simulink model "k1visproto"  (Simulink 8.2)
settings: Solver=ode45  StartTime=0.0  StopTime=10.0  RelTol=1e-3
libraries: cdsFiltCtrl x82, cdsFilt x45, cdsMuxMatrix x18, cdsEpicsOut x7, cdsEpicsBinIn x2, cdsAdcx0 x1, cdsAdcx1 x1, dac x1, simulink x1, cdsParameters x1
(part 14 of 14)

== system k1visproto/PROTO/TM/SERVOF ==
  L_IN : Inport
  P_IN : Inport  Port=2
  Y_IN : Inport  Port=3
  Ground1 : Ground
  Ground5 : Ground
  Ground6 : Ground
  L : cdsFiltCtrl/IIR FM with control  Tag=cdsFiltCtrl  Description=|
      | cdsFiltCntrl is the standard IIR filter module (exactly the same as cdsFilt) but with added control data output 'Ctrl'. Filter module digital signal output appears on the first output, which is called 'Val'. 'Ctrl' output has a bit pattern encoding the state of filter's on/off switches (FM1 through FM10). The bit values are:
      |                                                                                                                                                                                                                                                                                                                                       
      | module 	hex	dec                                                                                                                                                                                                                                                                                                                       
      | -----------------------                                                                                                                                                                                                                                                                                                               
      | FM1	0x20                    32                                                                                                                                                                                                                                                                                                        
      | FM2	0x80                     128                                                                                                                                                                                                                                                                                                      
      | FM3	0x200                   512                                                                                                                                                                                                                                                                                                       
      | FM4	0x800                   2048                                                                                                                                                                                                                                                                                                      
      | FM5	0x2000                 8192                                                                                                                                                                                                                                                                                                       
      | FM6	0x8000                 32768                                                                                                                                                                                                                                                                                                      
      | FM7	0x20000                131072                                                                                                                                                                                                                                                                                                     
      | FM8	0x80000                 524288                                                                                                                                                                                                                                                                                                    
      | FM9	0x200000               2097152                                                                                                                                                                                                                                                                                                    
      | FM10	0x800000               8388608                                                                                                                                                                                                                                                                                                   
      |                                                                                                                                                                                                                                                                                                                                       
      | This bit data can be used to drive some other switches or it can be output using a binary I/O module.
      settings: AttributesFormatString=%<Tag>
  P : cdsFiltCtrl/IIR FM with control  Tag=cdsFiltCtrl  Description=|
      | cdsFiltCntrl is the standard IIR filter module (exactly the same as cdsFilt) but with added control data output 'Ctrl'. Filter module digital signal output appears on the first output, which is called 'Val'. 'Ctrl' output has a bit pattern encoding the state of filter's on/off switches (FM1 through FM10). The bit values are:
      |                                                                                                                                                                                                                                                                                                                                       
      | module 	hex	dec                                                                                                                                                                                                                                                                                                                       
      | -----------------------                                                                                                                                                                                                                                                                                                               
      | FM1	0x20                    32                                                                                                                                                                                                                                                                                                        
      | FM2	0x80                     128                                                                                                                                                                                                                                                                                                      
      | FM3	0x200                   512                                                                                                                                                                                                                                                                                                       
      | FM4	0x800                   2048                                                                                                                                                                                                                                                                                                      
      | FM5	0x2000                 8192                                                                                                                                                                                                                                                                                                       
      | FM6	0x8000                 32768                                                                                                                                                                                                                                                                                                      
      | FM7	0x20000                131072                                                                                                                                                                                                                                                                                                     
      | FM8	0x80000                 524288                                                                                                                                                                                                                                                                                                    
      | FM9	0x200000               2097152                                                                                                                                                                                                                                                                                                    
      | FM10	0x800000               8388608                                                                                                                                                                                                                                                                                                   
      |                                                                                                                                                                                                                                                                                                                                       
      | This bit data can be used to drive some other switches or it can be output using a binary I/O module.
      settings: AttributesFormatString=%<Tag>
  Terminator1 : Terminator
  Terminator5 : Terminator
  Terminator6 : Terminator
  Y : cdsFiltCtrl/IIR FM with control  Tag=cdsFiltCtrl  Description=|
      | cdsFiltCntrl is the standard IIR filter module (exactly the same as cdsFilt) but with added control data output 'Ctrl'. Filter module digital signal output appears on the first output, which is called 'Val'. 'Ctrl' output has a bit pattern encoding the state of filter's on/off switches (FM1 through FM10). The bit values are:
      |                                                                                                                                                                                                                                                                                                                                       
      | module 	hex	dec                                                                                                                                                                                                                                                                                                                       
      | -----------------------                                                                                                                                                                                                                                                                                                               
      | FM1	0x20                    32                                                                                                                                                                                                                                                                                                        
      | FM2	0x80                     128                                                                                                                                                                                                                                                                                                      
      | FM3	0x200                   512                                                                                                                                                                                                                                                                                                       
      | FM4	0x800                   2048                                                                                                                                                                                                                                                                                                      
      | FM5	0x2000                 8192                                                                                                                                                                                                                                                                                                       
      | FM6	0x8000                 32768                                                                                                                                                                                                                                                                                                      
      | FM7	0x20000                131072                                                                                                                                                                                                                                                                                                     
      | FM8	0x80000                 524288                                                                                                                                                                                                                                                                                                    
      | FM9	0x200000               2097152                                                                                                                                                                                                                                                                                                    
      | FM10	0x800000               8388608                                                                                                                                                                                                                                                                                                   
      |                                                                                                                                                                                                                                                                                                                                       
      | This bit data can be used to drive some other switches or it can be output using a binary I/O module.
      settings: AttributesFormatString=%<Tag>
  L_Out : Outport
  P_Out : Outport  Port=2
  Y_Out : Outport  Port=3
  wires:
  Y/1 -> Y_Out/1
  P/1 -> P_Out/1
  Y_IN/1 -> Y/1
  Ground6/1 -> Y/2
  Y/2 -> Terminator6/1
  P_IN/1 -> P/1
  Ground5/1 -> P/2
  P/2 -> Terminator5/1
  L/1 -> L_Out/1
  L_IN/1 -> L/1
  Ground1/1 -> L/2
  L/2 -> Terminator1/1

== system k1visproto/PROTO/TM/TEST ==
  Ground1 : Ground
  Ground5 : Ground
  Ground6 : Ground
  L : cdsFilt/Subsystem  Tag=cdsFilt  Description=|
      | Purpose:                                                                                                                                                                                                                                  
      | Standard CDS IIR filter module.                                                                                                                                                                                                           
      |                                                                                                                                                                                                                                           
      | Operation:                                                                                                                                                                                                                                
      | Consists of 10 second order section IIR filters, plus a ramped gain stage. In FE code, also provides pre-defined test points and excitation channel inputs. The filter coefficients are defined in the LIGO system using the 'foton' tool.
      |                                                                                                                                                                                                                                           
      | Usage:                                                                                                                                                                                                                                    
      | Name the part with the desired filter module name.
      settings: AttributesFormatString=%<Tag>
  P : cdsFilt/Subsystem  Tag=cdsFilt  Description=|
      | Purpose:                                                                                                                                                                                                                                  
      | Standard CDS IIR filter module.                                                                                                                                                                                                           
      |                                                                                                                                                                                                                                           
      | Operation:                                                                                                                                                                                                                                
      | Consists of 10 second order section IIR filters, plus a ramped gain stage. In FE code, also provides pre-defined test points and excitation channel inputs. The filter coefficients are defined in the LIGO system using the 'foton' tool.
      |                                                                                                                                                                                                                                           
      | Usage:                                                                                                                                                                                                                                    
      | Name the part with the desired filter module name.
      settings: AttributesFormatString=%<Tag>
  Y : cdsFilt/Subsystem  Tag=cdsFilt  Description=|
      | Purpose:                                                                                                                                                                                                                                  
      | Standard CDS IIR filter module.                                                                                                                                                                                                           
      |                                                                                                                                                                                                                                           
      | Operation:                                                                                                                                                                                                                                
      | Consists of 10 second order section IIR filters, plus a ramped gain stage. In FE code, also provides pre-defined test points and excitation channel inputs. The filter coefficients are defined in the LIGO system using the 'foton' tool.
      |                                                                                                                                                                                                                                           
      | Usage:                                                                                                                                                                                                                                    
      | Name the part with the desired filter module name.
      settings: AttributesFormatString=%<Tag>
  L_Out : Outport
  P_Out : Outport  Port=2
  Y_Out : Outport  Port=3
  wires:
  Ground6/1 -> Y/1
  Ground5/1 -> P/1
  P/1 -> P_Out/1
  Y/1 -> Y_Out/1
  Ground1/1 -> L/1
  L/1 -> L_Out/1
